simulink model "ctrl_TT_ad_ctrl_cpp_ros_feedback"  (R2022b)
settings: Solver=FixedStepAuto  StartTime=0.0  StopTime=Tf  FixedStep=0.05  RelTol=1e-3
StopFcn:
  | save('testdata')
values from neighbouring files (symbols this model uses):
  adap = 1    [testdata.mat]
  Ba_0 = [0 0 0 0 0 0]    [testdata.mat]
  Bb = 4418825.3321    [testdata.mat]
  Bv_0 = [-5.14444 0 0 0 0 0]    [testdata.mat]
  Bx_0 = [70.34790039 -18.70597267 -370.8000183 0 0 0]    [testdata.mat]
  Cp = [-70.34790039 18.70597267 -370.8000183 -33.25566673 18.72042656 -369.9571533 3.8263092 17.99342728 -368.5174255 40.77630615 14.78142262 -366.2670288 ... (183 elements, 3x61)]    [testdata.mat]    (also in tester.m = [Cpx'; Cpy'; Cpz'])
  Cp_prime = [4.4510680392 0.0017344668 0.1011438 4.44985762706 -0.08575700726 0.1715736104 4.43452754992 -0.37550053768 0.2668049284 4.4276356638 -0.45576590634 0.3213246444 ... (183 elements, 3x61)]    [testdata.mat]
  d = 250    [testdata.mat]
  dA_BP1 = [0.00388591051125 0.00354364911083 0.00553040741788 0.00502167988714 0.0078585088908 0.00748424955325 0.0119232766011 0.0109054787122 0.0168329706434 0.016985509009 0.0156802934897 0.014556760782 ... (616 elements, 616x1)]    [testdata.mat]
  dA_BP2 = [0.00388594063171 0.00354357191533 0.00553040491113 0.00502170939051 0.00785855989083 0.00748435285791 0.0119232653011 0.0109054419481 0.0168329955973 0.0169854794658 0.015680230324 0.0145567225609 ... (616 elements, 616x1)]    [testdata.mat]
  dA_Hull = [0.896301676511 0.898896720864 0.884294141897 0.886832830172 0.870887902011 0.873360353662 0.856223658523 0.858613244346 0.840314828191 0.842595287849 0.823129385532 0.8253007603 ... (2914 elements, 2914x1)]    [testdata.mat]
  dA_PH = [0.00917454029683 0.00917454029683 0.00646521761836 0.00644666811643 0.011728531678 0.0107683420972 0.0165186720105 0.0100399866209 0.0121147162203 0.00917369783051 0.00917369783051 0.00646462373197 ... (550 elements, 550x1)]    [testdata.mat]
  dA_Sail = [0.08073747293 0.0655437895785 0.0678199581962 0.211496702297 0.185444652254 0.10949647106 0.0763960001413 0.0735864235671 0.0440728222699 0.281106392154 0.32735958292 0.104041938486 ... (564 elements, 564x1)]    [testdata.mat]
  dA_SProot = [0.0225345452169 0.0247277274893 0.0225345452169 0.0480467976325 0.0166447079844 0.0410754287554 0.0247277274893 0.0480467976325 0.0468898715351 0.0839833312794 0.0166447079844 0.0255016718 ... (904 elements, 904x1)]    [testdata.mat]
  dA_X1a = [0.0149621011817 0.0166706156701 0.0341149781095 0.0355915100668 0.0512235531199 0.0489176133683 0.0604458424392 0.0503279152264 0.0577124835488 0.0401555322121 0.044833653096 0.0251568218541 ... (200 elements, 200x1)]    [testdata.mat]
  dA_X1b = [0.0149621011817 0.0166706156701 0.0341149781095 0.0355915100668 0.0512235531199 0.0489176133683 0.0604458424392 0.0503279152264 0.0577124835488 0.0401555322121 0.044833653096 0.0251568218541 ... (200 elements, 200x1)]    [testdata.mat]
  dA_X2a = [0.0149620639393 0.0166705502855 0.0341150948266 0.0355913495849 0.051223110376 0.0489180393921 0.0604458270347 0.0503275686692 0.0577128112225 0.0401556683139 0.0448334591683 0.0251566482124 ... (200 elements, 200x1)]    [testdata.mat]
  dA_X2b = [0.0149620639393 0.0166705502855 0.0341150948266 0.0355913495849 0.051223110376 0.0489180393921 0.0604458270347 0.0503275686692 0.0577128112225 0.0401556683139 0.0448334591683 0.0251566482124 ... (200 elements, 200x1)]    [testdata.mat]
  dA_X3a = [0.0149621011817 0.0166706156701 0.0341149781095 0.0355915100668 0.0512235531199 0.0489176133683 0.0604458424392 0.0503279152264 0.0577124835488 0.0401555322121 0.044833653096 0.0251568218541 ... (200 elements, 200x1)]    [testdata.mat]
  dA_X3b = [0.0149621011817 0.0166706156701 0.0341149781095 0.0355915100668 0.0512235531199 0.0489176133683 0.0604458424392 0.0503279152264 0.0577124835488 0.0401555322121 0.044833653096 0.0251568218541 ... (200 elements, 200x1)]    [testdata.mat]
  dA_X4a = [0.0149621011817 0.0166706156701 0.0341149781095 0.0355915100668 0.0512235531199 0.0489176133683 0.0604458424392 0.0503279152264 0.0577124835488 0.0401555322121 0.044833653096 0.0251568218541 ... (200 elements, 200x1)]    [testdata.mat]
  dA_X4b = [0.0149621011817 0.0166706156701 0.0341149781095 0.0355915100668 0.0512235531199 0.0489176133683 0.0604458424392 0.0503279152264 0.0577124835488 0.0401555322121 0.044833653096 0.0251568218541 ... (200 elements, 200x1)]    [testdata.mat]
  Ixx = 52300000    [testdata.mat]
  Ixy = 0    [testdata.mat]
  Ixz = 0    [testdata.mat]
  Iyy = 1375000000    [testdata.mat]
  Iyz = 0    [testdata.mat]
  Izz = 1367000000    [testdata.mat]
  Kp = 0.1    [testdata.mat]
  L1 =     [testdata.mat]
  Mb = 4418825.3321    [testdata.mat]
  n_BP1 = [-0.7747315 -0.03638153 -0.4095958 0 -0.1221389 0 -0.01670914 0 0.005209626 0 0.03404154 0 ... (1848 elements, 616x3)]    [testdata.mat]
  n_BP2 = [-0.774731517 -0.0363815315 -0.409595788 0 -0.122138903 0 -0.0167091396 0 0.00520962616 0 0.0340415388 0 ... (1848 elements, 616x3)]    [testdata.mat]
  n_Hull = [-3.334458e-05 -1.700098e-14 -3.354233e-05 -1.686235e-14 -3.289162e-05 -1.685701e-14 -3.291391e-05 -1.698144e-14 -3.338145e-05 -1.688959e-14 -3.29289e-05 -1.682536e-14 ... (8742 elements, 2914x3)]    [testdata.mat]
  n_PH = [0 0 0.01711651 0.01711627 0.2676807 0.2676804 0.7675173 0.7675174 0.9857236 0 0 0.01711456 ... (1650 elements, 550x3)]    [testdata.mat]
  n_Sail = [-0.05126832 -0.05168081 -0.0485872 -0.03288998 -0.03203588 -0.04435105 -0.04335441 -0.04419429 -0.05169604 0.01094904 0.01649325 -0.03825178 ... (1692 elements, 564x3)]    [testdata.mat]
  n_SProot = [-0.7837688 -0.7969784 -0.7837688 -0.79448 -0.280412 -0.3378876 -0.7969784 -0.79448 -0.7910827 -0.3483897 -0.280412 -0.2790298 ... (2712 elements, 904x3)]    [testdata.mat]
  n_X2a = [-0.283297986 -0.283136904 -0.283195704 -0.28313759 -0.2831586 -0.283137113 -0.28313911 -0.283136606 -0.283121586 -0.283136815 -0.283108413 -0.283138901 ... (600 elements, 200x3)]    [testdata.mat]
  n_X2b = [-0.283297986 -0.283136904 -0.283195704 -0.28313759 -0.2831586 -0.283137113 -0.28313911 -0.283136606 -0.283121586 -0.283136815 -0.283108413 -0.283138901 ... (600 elements, 200x3)]    [testdata.mat]
  n_X3a = [-0.283298 -0.2831369 -0.2831957 -0.2831376 -0.2831586 -0.2831371 -0.2831391 -0.2831366 -0.2831216 -0.2831368 -0.2831084 -0.2831389 ... (600 elements, 200x3)]    [testdata.mat]
  n_X4a = [-0.283298 -0.2831369 -0.2831957 -0.2831376 -0.2831586 -0.2831371 -0.2831391 -0.2831366 -0.2831216 -0.2831368 -0.2831084 -0.2831389 ... (600 elements, 200x3)]    [testdata.mat]
  n_X4b = [-0.283298 -0.2831369 -0.2831957 -0.2831376 -0.2831586 -0.2831371 -0.2831391 -0.2831366 -0.2831216 -0.2831368 -0.2831084 -0.2831389 ... (600 elements, 200x3)]    [testdata.mat]
  nt_BP1 = 616    [testdata.mat]
  nt_BP2 = 616    [testdata.mat]
  nt_Hull = 2914    [testdata.mat]
  nt_PH = 550    [testdata.mat]
  nt_Sail = 564    [testdata.mat]
  nt_SProot = 904    [testdata.mat]
  nt_X1a = 200    [testdata.mat]
  nt_X1b = 200    [testdata.mat]
  nt_X2a = 200    [testdata.mat]
  nt_X2b = 200    [testdata.mat]
  nt_X3a = 200    [testdata.mat]
  nt_X3b = 200    [testdata.mat]
  nt_X4a = 200    [testdata.mat]
  nt_X4b = 200    [testdata.mat]
  Seastate = 0    [testdata.mat]
  Tf = 500    [testdata.mat]    (also in tester.m)
  Ts = 0.05    [testdata.mat]
  vt1_BP1 = [-11.0524049722 -10.9924120522 -10.9924120522 -10.8819663922 -10.8819663922 -10.7297166322 -10.7297166322 -10.5070632922 -10.5070632922 -10.1807245522 -10.1807245522 -9.8815181122 ... (1848 elements, 616x3)]    [testdata.mat]
  vt1_BP2 = [-11.0524048318 -10.9924111396 -10.9924111396 -10.8819658306 -10.8819658306 -10.7297157898 -10.7297157898 -10.5070637134 -10.5070637134 -10.1807238502 -10.1807238502 -9.8815188844 ... (1848 elements, 616x3)]    [testdata.mat]
  vt1_Hull = [3.5122487678 3.7304022878 5.2621803278 5.4863499878 6.9866994878 7.2167238278 8.6832650078 8.9189474678 10.3493567078 10.5904445678 11.9823842078 12.2286247478 ... (8742 elements, 2914x3)]    [testdata.mat]
  vt1_PH = [37.3342788278 37.3342788278 37.4268866678 37.4268866678 37.5892452278 37.5892452278 37.7549453078 37.7549453078 37.8074619278 37.3342788278 37.3342788278 37.4268866678 ... (1650 elements, 550x3)]    [testdata.mat]
  vt1_Sail = [-12.4909433722 -12.1578443722 -12.0399645322 -11.2138368922 -10.6240515922 -11.5111900522 -11.9364967522 -11.6561249722 -12.4909433722 -7.5732648922 -6.8453119522 -11.1890071522 ... (1692 elements, 564x3)]    [testdata.mat]
  vt1_SProot = [29.2099766678 29.1371231078 29.0494854278 29.2099766678 29.2862630078 29.4526510478 29.0494854278 29.1261368078 29.3369263478 29.5706712878 29.0494854278 29.3857364078 ... (2712 elements, 904x3)]    [testdata.mat]
  vt1_X1a = [29.3961751478 29.4776282078 29.4776282078 29.7060309278 29.7060309278 30.0693861278 30.0693861278 30.5458756478 30.5458756478 31.0830460478 31.0830460478 31.6023926678 ... (600 elements, 200x3)]    [testdata.mat]
  vt1_X1b = [29.6638337078 29.6638337078 29.9620713878 29.9620713878 30.3181187678 30.3181187678 30.7116389078 30.7116389078 31.1104380878 31.1104380878 31.4810519678 31.4810519678 ... (600 elements, 200x3)]    [testdata.mat]
  vt1_X2a = [29.3961767624 29.4776272952 29.4776272952 29.7060326828 29.7060326828 30.0693842324 30.0693842324 30.5458736822 30.5458736822 31.083047171 31.083047171 31.6023916148 ... (600 elements, 200x3)]    [testdata.mat]
  vt1_X2b = [29.6638345502 29.6638345502 29.9620708964 29.9620708964 30.3181168022 30.3181168022 30.7116409436 30.7116409436 31.1104372454 31.1104372454 31.4810526698 31.4810526698 ... (600 elements, 200x3)]    [testdata.mat]
  vt1_X3a = [29.3961751478 29.4776282078 29.4776282078 29.7060309278 29.7060309278 30.0693861278 30.0693861278 30.5458756478 30.5458756478 31.0830460478 31.0830460478 31.6023926678 ... (600 elements, 200x3)]    [testdata.mat]
  vt1_X3b = [29.6638337078 29.6638337078 29.9620713878 29.9620713878 30.3181187678 30.3181187678 30.7116389078 30.7116389078 31.1104380878 31.1104380878 31.4810519678 31.4810519678 ... (600 elements, 200x3)]    [testdata.mat]
  vt1_X4a = [29.6638337078 29.6638337078 29.9620713878 29.9620713878 30.3181187678 30.3181187678 30.7116389078 30.7116389078 31.1104380878 31.1104380878 31.4810519678 31.4810519678 ... (600 elements, 200x3)]    [testdata.mat]
  vt1_X4b = [29.3961751478 29.4776282078 29.4776282078 29.7060309278 29.7060309278 30.0693861278 30.0693861278 30.5458756478 30.5458756478 31.0830460478 31.0830460478 31.6023926678 ... (600 elements, 200x3)]    [testdata.mat]
  vt2_BP1 = [-10.9924120522 -10.9494777322 -10.8819663922 -10.8505308322 -10.7297166322 -10.7112259522 -10.5070632922 -10.4997203722 -10.1807245522 -10.1757543922 -9.8815181122 -9.8813004922 ... (1848 elements, 616x3)]    [testdata.mat]
  vt2_BP2 = [-11.0294626294 -11.0294626294 -10.9494786448 -10.9494786448 -10.8505316746 -10.8505316746 -10.7112256012 -10.7112256012 -10.499720302 -10.499720302 -10.1757550942 -10.1757550942 ... (1848 elements, 616x3)]    [testdata.mat]
  vt2_Hull = [1.9517168078 1.9517168078 3.7304022878 3.7304022878 5.4863499878 5.4863499878 7.2167238278 7.2167238278 8.9189474678 8.9189474678 10.5904445678 10.5904445678 ... (8742 elements, 2914x3)]    [testdata.mat]
  vt2_PH = [37.2028433678 37.2028433678 37.3342788278 37.4268866678 37.4268866678 37.5892452278 37.5892452278 37.7549453078 37.7549453078 37.2028433678 37.2028433678 37.3342788278 ... (1650 elements, 550x3)]    [testdata.mat]
  vt2_Sail = [-12.0399645322 -12.0399645322 -11.9364967522 -10.7084881522 -10.7084881522 -12.0399645322 -12.0399645322 -11.9364967522 -12.3734566522 -7.7110323922 -7.7110323922 -11.6561249722 ... (1692 elements, 564x3)]    [testdata.mat]
  vt2_SProot = [29.0494854278 29.0494854278 29.2099766678 29.1261368078 29.0494854278 29.1371231078 29.1371231078 29.2099766678 29.1261368078 29.2099766678 29.2862630078 29.2862630078 ... (2712 elements, 904x3)]    [testdata.mat]
  vt2_X1a = [29.4776282078 29.9620713878 29.7060309278 30.3181187678 30.0693861278 30.7116389078 30.5458756478 31.1104380878 31.0830460478 31.4810519678 31.6023926678 31.7970362078 ... (600 elements, 200x3)]    [testdata.mat]
  vt2_X1b = [29.4776282078 29.9620713878 29.7060309278 30.3181187678 30.0693861278 30.7116389078 30.5458756478 31.1104380878 31.0830460478 31.4810519678 31.6023926678 31.7970362078 ... (600 elements, 200x3)]    [testdata.mat]
  vt2_X2a = [29.6638345502 29.6638345502 29.9620708964 29.9620708964 30.3181168022 30.3181168022 30.7116409436 30.7116409436 31.1104372454 31.1104372454 31.4810526698 31.4810526698 ... (600 elements, 200x3)]    [testdata.mat]
  vt2_X2b = [29.3961767624 29.4776272952 29.4776272952 29.7060326828 29.7060326828 30.0693842324 30.0693842324 30.5458736822 30.5458736822 31.083047171 31.083047171 31.6023916148 ... (600 elements, 200x3)]    [testdata.mat]
  vt2_X3a = [29.4776282078 29.9620713878 29.7060309278 30.3181187678 30.0693861278 30.7116389078 30.5458756478 31.1104380878 31.0830460478 31.4810519678 31.6023926678 31.7970362078 ... (600 elements, 200x3)]    [testdata.mat]
  vt2_X3b = [29.4776282078 29.9620713878 29.7060309278 30.3181187678 30.0693861278 30.7116389078 30.5458756478 31.1104380878 31.0830460478 31.4810519678 31.6023926678 31.7970362078 ... (600 elements, 200x3)]    [testdata.mat]
  vt2_X4a = [29.4776282078 29.9620713878 29.7060309278 30.3181187678 30.0693861278 30.7116389078 30.5458756478 31.1104380878 31.0830460478 31.4810519678 31.6023926678 31.7970362078 ... (600 elements, 200x3)]    [testdata.mat]
  vt2_X4b = [29.4776282078 29.9620713878 29.7060309278 30.3181187678 30.0693861278 30.7116389078 30.5458756478 31.1104380878 31.0830460478 31.4810519678 31.6023926678 31.7970362078 ... (600 elements, 200x3)]    [testdata.mat]
  vt3_BP1 = [-11.0294636122 -11.0294636122 -10.9494777322 -10.9494777322 -10.8505308322 -10.8505308322 -10.7112259522 -10.7112259522 -10.4997203722 -10.4997203722 -10.1757543922 -10.1757543922 ... (1848 elements, 616x3)]    [testdata.mat]
  vt3_BP2 = [-10.9924111396 -10.9494786448 -10.8819658306 -10.8505316746 -10.7297157898 -10.7112256012 -10.5070637134 -10.499720302 -10.1807238502 -10.1757550942 -9.8815188844 -9.8813013346 ... (1848 elements, 616x3)]    [testdata.mat]
  vt3_Hull = [1.7397198278 3.5122487678 3.5122487678 5.2621803278 5.2621803278 6.9866994878 6.9866994878 8.6832650078 8.6832650078 10.3493567078 10.3493567078 11.9823842078 ... (8742 elements, 2914x3)]    [testdata.mat]
  vt3_PH = [37.2028433678 37.3342788278 37.3342788278 37.3342788278 37.4268866678 37.4268866678 37.5892452278 37.5892452278 37.7549453078 37.2028433678 37.3342788278 37.3342788278 ... (1650 elements, 550x3)]    [testdata.mat]
  vt3_Sail = [-12.3734566522 -12.4909433722 -12.3734566522 -11.5111900522 -11.2138368922 -11.7698559922 -11.5111900522 -11.5111900522 -12.1578443722 -8.3109054322 -7.5732648922 -11.5111900522 ... (1692 elements, 564x3)]    [testdata.mat]
  vt3_SProot = [29.1261368078 29.2099766678 29.1261368078 29.3369263478 29.1371231078 29.2099766678 29.2099766678 29.3369263478 29.2548344678 29.3369263478 29.1371231078 29.1371231078 ... (2712 elements, 904x3)]    [testdata.mat]
  vt3_X1a = [29.6638337078 29.6638337078 29.9620713878 29.9620713878 30.3181187678 30.3181187678 30.7116389078 30.7116389078 31.1104380878 31.1104380878 31.4810519678 31.4810519678 ... (600 elements, 200x3)]    [testdata.mat]
  vt3_X1b = [29.3961751478 29.4776282078 29.4776282078 29.7060309278 29.7060309278 30.0693861278 30.0693861278 30.5458756478 30.5458756478 31.0830460478 31.0830460478 31.6023926678 ... (600 elements, 200x3)]    [testdata.mat]
  vt3_X2a = [29.4776272952 29.9620708964 29.7060326828 30.3181168022 30.0693842324 30.7116409436 30.5458736822 31.1104372454 31.083047171 31.4810526698 31.6023916148 31.7970343826 ... (600 elements, 200x3)]    [testdata.mat]
  vt3_X2b = [29.4776272952 29.9620708964 29.7060326828 30.3181168022 30.0693842324 30.7116409436 30.5458736822 31.1104372454 31.083047171 31.4810526698 31.6023916148 31.7970343826 ... (600 elements, 200x3)]    [testdata.mat]
  vt3_X3a = [29.6638337078 29.6638337078 29.9620713878 29.9620713878 30.3181187678 30.3181187678 30.7116389078 30.7116389078 31.1104380878 31.1104380878 31.4810519678 31.4810519678 ... (600 elements, 200x3)]    [testdata.mat]
  vt3_X3b = [29.3961751478 29.4776282078 29.4776282078 29.7060309278 29.7060309278 30.0693861278 30.0693861278 30.5458756478 30.5458756478 31.0830460478 31.0830460478 31.6023926678 ... (600 elements, 200x3)]    [testdata.mat]
  vt3_X4a = [29.3961751478 29.4776282078 29.4776282078 29.7060309278 29.7060309278 30.0693861278 30.0693861278 30.5458756478 30.5458756478 31.0830460478 31.0830460478 31.6023926678 ... (600 elements, 200x3)]    [testdata.mat]
  vt3_X4b = [29.6638337078 29.6638337078 29.9620713878 29.9620713878 30.3181187678 30.3181187678 30.7116389078 30.7116389078 31.1104380878 31.1104380878 31.4810519678 31.4810519678 ... (600 elements, 200x3)]    [testdata.mat]
  Xb = 0    [testdata.mat]
  Xcg = [32.3287332922 0 0]    [testdata.mat]
  Xg = 0    [testdata.mat]
  Yb = 0    [testdata.mat]
  Yg = 0    [testdata.mat]
  Zb = 0.4406    [testdata.mat]
  Zg = 0    [testdata.mat]
libraries: robotlib x54, simulink x8, sharedtransform x2, dspmathops x2
(part 1 of 9)
settings Model: Creator=yagkim  LastModifiedBy=vpetrov
settings SolverCC: AlgebraicLoopSolver=TrustRegion
settings OptimizationCC: EnhancedBackFolding=on  PassReuseOutputArgsAs=Individual arguments  ZeroExternalMemoryAtStartup=off  ZeroInternalMemoryAtStartup=off  MaxStackSize=64  OptimizeBlockOrder=speed  DifferentSizesBufferReuse=on  OptimizationCustomize=off  EfficientTunableParamExpr=on
settings DebuggingCC: ParameterTunabilityLossMsg=error  UnconnectedInputMsg=warning  UnconnectedOutputMsg=warning  UnconnectedLineMsg=warning  SFMachineParentedDataDiag=warning  ArithmeticOperatorsInVariantConditions=warning
settings HardwareCC: ProdBitPerPointer=32  ProdBitPerSizeT=32  ProdBitPerPtrDiffT=32  ProdLargestAtomicFloat=None  ProdIntDivRoundTo=Undefined  ProdEndianess=Unspecified  ProdWordSize=32  ProdHWDeviceType=Generic->Unspecified (assume 32-bit Generic)
settings ModelReferenceCC: EnableRefExpFcnMdlSchedulingChecks=on
settings SFSimCC: MATLABDynamicMemAlloc=off  CustomCodeUndefinedFunction=UseInterfaceOnly  SimTargetLang=C++
settings RTWCC: Description=Embedded Coder  SystemTargetFile=ert.tlc  HardwareBoard=Robot Operating System (ROS)  TLCOptions="-aInlineSetEventsForThisBaseRateFcn=TLC_FALSE -aSuppressMultiTaskScheduler=TLC_FALSE  -aRateBasedStepFcn=0"  TemplateMakefile=ert_default_tmf  GenerateReport=on  Toolchain=Catkin  LaunchReport=on  TargetLang=C++  DLArmComputeVersion=19.05
settings CodeAppCC: ForceParamTrailComments=on  IgnoreCustomStorageClasses=off  OperatorAnnotations=on  SimulinkDataObjDesc=on  SFDataObjDesc=on  InsertBlockDesc=on
settings ERTTargetCC: SupportContinuousTime=on

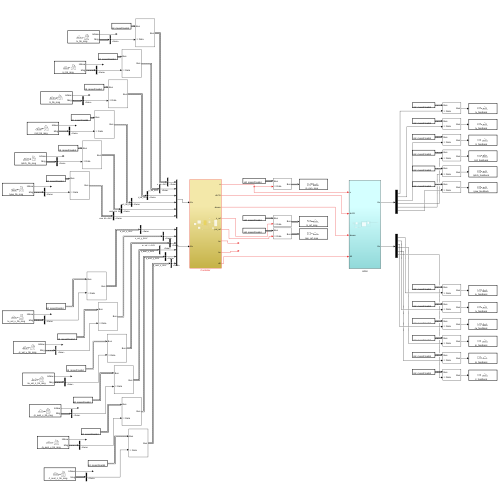
[thumbnail: Simulink's stored preview of the top-level diagram]
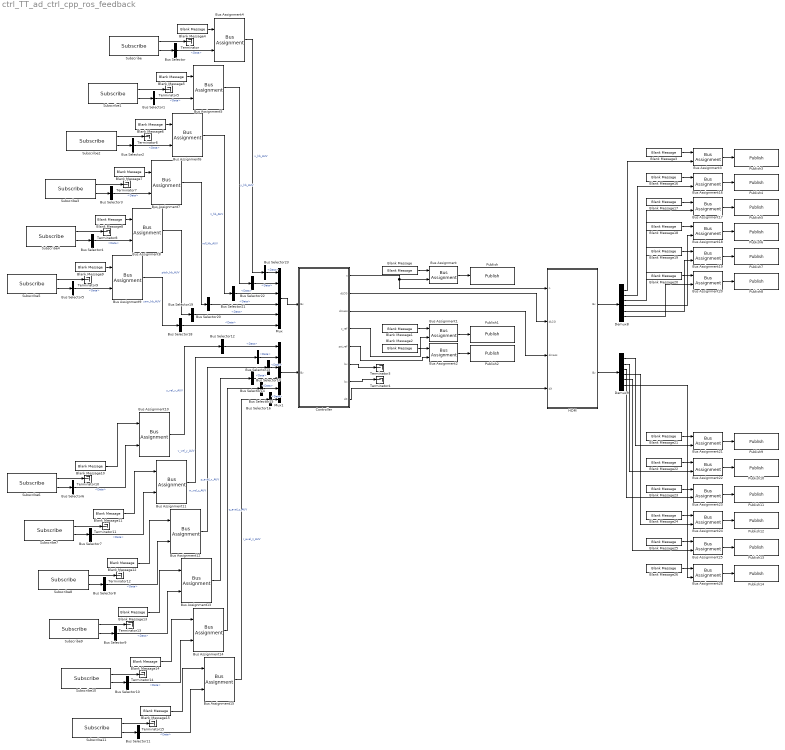
== system ctrl_TT_ad_ctrl_cpp_ros_feedback ==
  Blank Message{,1..26} (27 alike) : robotlib/Blank Message  messageClass=Message  entityType=std_msgs/Float64  messageType=std_msgs/Float64  SampleTime=inf  legacyBusStruct=off
      settings: LibrarySourceBlock=roslib/ROS/Blank Message
  Bus Assignment{,1..26} (27 alike) : BusAssignment  AssignedSignals=Data
  Bus Selector{,1..23} (24 alike) : BusSelector  OutputSignals=Data
  Controller : Subsystem
  Demux8 : Demux  Outputs=6
  Demux9 : Demux  Outputs=6
  HDM : Subsystem
  Mux : Mux  Inputs=6
  Mux1 : Mux  Inputs=6
  Publish : robotlib/Publish  topicSource=Specify your own  topic=/n_rpm_msg  messageType=std_msgs/Float64  legacyBusStruct=off  messageQueueLength=1
      settings: LibrarySourceBlock=roslib/ROS/Publish
  Publish1 : robotlib/Publish  topicSource=Specify your own  topic=/z_ref_msg  messageType=std_msgs/Float64  legacyBusStruct=off  messageQueueLength=1
      settings: LibrarySourceBlock=roslib/ROS/Publish
  Publish10 : robotlib/Publish  topicSource=Specify your own  topic=/v_feedback  messageType=std_msgs/Float64  legacyBusStruct=off  messageQueueLength=1
      settings: LibrarySourceBlock=roslib/ROS/Publish
  Publish11 : robotlib/Publish  topicSource=Specify your own  topic=/w_feedback  messageType=std_msgs/Float64  legacyBusStruct=off  messageQueueLength=1
      settings: LibrarySourceBlock=roslib/ROS/Publish
  Publish12 : robotlib/Publish  topicSource=Specify your own  topic=/p_feedback  messageType=std_msgs/Float64  legacyBusStruct=off  messageQueueLength=1
      settings: LibrarySourceBlock=roslib/ROS/Publish
  Publish13 : robotlib/Publish  topicSource=Specify your own  topic=/q_feedback  messageType=std_msgs/Float64  legacyBusStruct=off  messageQueueLength=1
      settings: LibrarySourceBlock=roslib/ROS/Publish
  Publish14 : robotlib/Publish  topicSource=Specify your own  topic=/r_feedback  messageType=std_msgs/Float64  legacyBusStruct=off  messageQueueLength=1
      settings: LibrarySourceBlock=roslib/ROS/Publish
  Publish2 : robotlib/Publish  topicSource=Specify your own  topic=/psi_ref_msg  messageType=std_msgs/Float64  legacyBusStruct=off  messageQueueLength=1
      settings: LibrarySourceBlock=roslib/ROS/Publish
  Publish3 : robotlib/Publish  topicSource=Specify your own  topic=/x_feedback  messageType=std_msgs/Float64  legacyBusStruct=off  messageQueueLength=1
      settings: LibrarySourceBlock=roslib/ROS/Publish
  Publish4 : robotlib/Publish  topicSource=Specify your own  topic=/y_feedback  messageType=std_msgs/Float64  legacyBusStruct=off  messageQueueLength=1
      settings: LibrarySourceBlock=roslib/ROS/Publish
  Publish5 : robotlib/Publish  topicSource=Specify your own  topic=/z_feedback  messageType=std_msgs/Float64  legacyBusStruct=off  messageQueueLength=1
      settings: LibrarySourceBlock=roslib/ROS/Publish
  Publish6 : robotlib/Publish  topicSource=Specify your own  topic=/roll_feedback  messageType=std_msgs/Float64  legacyBusStruct=off  messageQueueLength=1
      settings: LibrarySourceBlock=roslib/ROS/Publish
  Publish7 : robotlib/Publish  topicSource=Specify your own  topic=/pitch_feedback  messageType=std_msgs/Float64  legacyBusStruct=off  messageQueueLength=1
      settings: LibrarySourceBlock=roslib/ROS/Publish
  Publish8 : robotlib/Publish  topicSource=Specify your own  topic=/yaw_feedback  messageType=std_msgs/Float64  legacyBusStruct=off  messageQueueLength=1
      settings: LibrarySourceBlock=roslib/ROS/Publish
  Publish9 : robotlib/Publish  topicSource=Specify your own  topic=/u_feedback  messageType=std_msgs/Float64  legacyBusStruct=off  messageQueueLength=1
      settings: LibrarySourceBlock=roslib/ROS/Publish
  Subscribe : robotlib/Subscribe  topicSource=Specify your own  topic=/x_hb_msg  messageType=std_msgs/Float64  SampleTime=-1  legacyBusStruct=off  messageQueueLength=1
      settings: LibrarySourceBlock=roslib/ROS/Subscribe
  Subscribe1 : robotlib/Subscribe  topicSource=Specify your own  topic=/y_hb_msg  messageType=std_msgs/Float64  SampleTime=-1  legacyBusStruct=off  messageQueueLength=1
      settings: LibrarySourceBlock=roslib/ROS/Subscribe
  Subscribe10 : robotlib/Subscribe  topicSource=Specify your own  topic=/q_avel_y_hb_msg  messageType=std_msgs/Float64  SampleTime=-1  legacyBusStruct=off  messageQueueLength=1
      settings: LibrarySourceBlock=roslib/ROS/Subscribe
  Subscribe11 : robotlib/Subscribe  topicSource=Specify your own  topic=/r_avel_z_hb_msg  messageType=std_msgs/Float64  SampleTime=-1  legacyBusStruct=off  messageQueueLength=1
      settings: LibrarySourceBlock=roslib/ROS/Subscribe
  Subscribe2 : robotlib/Subscribe  topicSource=Specify your own  topic=/z_hb_msg  messageType=std_msgs/Float64  SampleTime=-1  legacyBusStruct=off  messageQueueLength=1
      settings: LibrarySourceBlock=roslib/ROS/Subscribe
  Subscribe3 : robotlib/Subscribe  topicSource=Specify your own  topic=/roll_hb_msg  messageType=std_msgs/Float64  SampleTime=-1  legacyBusStruct=off  messageQueueLength=1
      settings: LibrarySourceBlock=roslib/ROS/Subscribe
  Subscribe4 : robotlib/Subscribe  topicSource=Specify your own  topic=/pitch_hb_msg  messageType=std_msgs/Float64  SampleTime=-1  legacyBusStruct=off  messageQueueLength=1
      settings: LibrarySourceBlock=roslib/ROS/Subscribe
  Subscribe5 : robotlib/Subscribe  topicSource=Specify your own  topic=/yaw_hb_msg  messageType=std_msgs/Float64  SampleTime=-1  legacyBusStruct=off  messageQueueLength=1
      settings: LibrarySourceBlock=roslib/ROS/Subscribe
  Subscribe6 : robotlib/Subscribe  topicSource=Specify your own  topic=/u_vel_x_hb_msg  messageType=std_msgs/Float64  SampleTime=-1  legacyBusStruct=off  messageQueueLength=1
      settings: LibrarySourceBlock=roslib/ROS/Subscribe
  Subscribe7 : robotlib/Subscribe  topicSource=Specify your own  topic=/v_vel_y_hb_msg  messageType=std_msgs/Float64  SampleTime=-1  legacyBusStruct=off  messageQueueLength=1
      settings: LibrarySourceBlock=roslib/ROS/Subscribe
  Subscribe8 : robotlib/Subscribe  topicSource=Specify your own  topic=/w_vel_z_hb_msg  messageType=std_msgs/Float64  SampleTime=-1  legacyBusStruct=off  messageQueueLength=1
      settings: LibrarySourceBlock=roslib/ROS/Subscribe
  Subscribe9 : robotlib/Subscribe  topicSource=Specify your own  topic=/p_avel_x_hb_msg  messageType=std_msgs/Float64  SampleTime=-1  legacyBusStruct=off  messageQueueLength=1
      settings: LibrarySourceBlock=roslib/ROS/Subscribe
  Terminator{,3..15} (14 alike) : Terminator
  wires:
  Bus Assignment4/1 -> Bus Selector23/1  "x_hb_AUV"
  Bus Assignment6/1 -> Bus Selector21/1  "z_hb_AUV"
  Bus Assignment7/1 -> Bus Selector20/1  "roll_hb_AUV"
  Bus Assignment8/1 -> Bus Selector19/1  "pitch_hb_AUV"
  Bus Assignment9/1 -> Bus Selector18/1  "yaw_hb_AUV"
  Mux/1 -> Controller/1(Bx)
  Mux1/1 -> Controller/2(Bv)
  Bus Assignment11/1 -> Bus Selector13/1  "v_vel_y_AUV"
  Bus Assignment12/1 -> Bus Selector17/1  "w_vel_z_AUV"
  Bus Assignment13/1 -> Bus Selector14/1  "p_avel_x_AUV"
  Bus Assignment14/1 -> Bus Selector15/1  "q_avel_y_AUV"
  Bus Assignment15/1 -> Bus Selector16/1  "r_avel_z_AUV"
  Controller/2(dLCG) -> HDM/2(dLCG)
  Controller/3(dmass) -> HDM/3(dmass)
  Controller/1(n) -> Bus Assignment/2, HDM/1(n)
  Controller/4(z_ref) -> Bus Assignment1/2
  Controller/5(psi_ref) -> Bus Assignment2/2
  Controller/6(bv) -> Terminator3/1
  Controller/7(bx) -> Terminator4/1
  Bus Assignment/1 -> Publish/1
  Blank Message/1 -> Bus Assignment/1
  Blank Message1/1 -> Bus Assignment1/1
  Bus Assignment1/1 -> Publish1/1
  Blank Message2/1 -> Bus Assignment2/1
  Bus Assignment2/1 -> Publish2/1
  Subscribe/1 -> Terminator/1
  Bus Selector/1 -> Bus Assignment4/2  "<Data>"
  Subscribe/2 -> Bus Selector/1
  Blank Message4/1 -> Bus Assignment4/1
  Subscribe1/1 -> Terminator5/1
  Bus Selector1/1 -> Bus Assignment5/2  "<Data>"
  Blank Message5/1 -> Bus Assignment5/1
  Subscribe1/2 -> Bus Selector1/1
  Bus Assignment5/1 -> Bus Selector22/1  "y_hb_AUV"
  Blank Message6/1 -> Bus Assignment6/1
  Bus Selector2/1 -> Bus Assignment6/2  "<Data>"
  Subscribe2/2 -> Bus Selector2/1
  Subscribe2/1 -> Terminator6/1
  Blank Message7/1 -> Bus Assignment7/1
  Bus Selector3/1 -> Bus Assignment7/2  "<Data>"
  Subscribe3/2 -> Bus Selector3/1
  Subscribe3/1 -> Terminator7/1
  Blank Message8/1 -> Bus Assignment8/1
  Bus Selector4/1 -> Bus Assignment8/2  "<Data>"
  Subscribe4/2 -> Bus Selector4/1
  Subscribe4/1 -> Terminator8/1
  Bus Selector5/1 -> Bus Assignment9/2  "<Data>"
  Subscribe5/2 -> Bus Selector5/1
  Blank Message9/1 -> Bus Assignment9/1
  Subscribe5/1 -> Terminator9/1
  Bus Selector6/1 -> Bus Assignment10/2  "<Data>"
  Subscribe6/2 -> Bus Selector6/1
  Blank Message10/1 -> Bus Assignment10/1
  Subscribe6/1 -> Terminator10/1
  Bus Assignment10/1 -> Bus Selector12/1  "u_vel_x_AUV"
  Bus Selector7/1 -> Bus Assignment11/2  "<Data>"
  Blank Message11/1 -> Bus Assignment11/1
  Subscribe7/2 -> Bus Selector7/1
  Subscribe7/1 -> Terminator11/1
  Bus Selector8/1 -> Bus Assignment12/2  "<Data>"
  Blank Message12/1 -> Bus Assignment12/1
  Subscribe8/2 -> Bus Selector8/1
  Subscribe8/1 -> Terminator12/1
  Bus Selector9/1 -> Bus Assignment13/2  "<Data>"
  Blank Message13/1 -> Bus Assignment13/1
  Subscribe9/2 -> Bus Selector9/1
  Subscribe9/1 -> Terminator13/1
  Bus Selector10/1 -> Bus Assignment14/2  "<Data>"
  Blank Message14/1 -> Bus Assignment14/1
  Subscribe10/2 -> Bus Selector10/1
  Subscribe10/1 -> Terminator14/1
  Bus Selector11/1 -> Bus Assignment15/2  "<Data>"
  Blank Message15/1 -> Bus Assignment15/1
  Subscribe11/2 -> Bus Selector11/1
  Subscribe11/1 -> Terminator15/1
  Bus Selector12/1 -> Mux1/1  "<Data>"
  Bus Selector13/1 -> Mux1/2  "<Data>"
  Bus Selector14/1 -> Mux1/4  "<Data>"
  Bus Selector15/1 -> Mux1/5  "<Data>"
  Bus Selector16/1 -> Mux1/6  "<Data>"
  Bus Selector17/1 -> Mux1/3  "<Data>"
  Bus Selector18/1 -> Mux/6  "<Data>"
  Bus Selector19/1 -> Mux/5  "<Data>"
  Bus Selector20/1 -> Mux/4  "<Data>"
  Bus Selector21/1 -> Mux/3  "<Data>"
  Bus Selector22/1 -> Mux/2  "<Data>"
  Bus Selector23/1 -> Mux/1  "<Data>"
  Controller/8(dX) -> HDM/4(dX)
  HDM/1(Bx) -> Demux8/1
  HDM/2(Bv) -> Demux9/1
  Blank Message3/1 -> Bus Assignment3/1
  Demux8/1 -> Bus Assignment3/2
  Bus Assignment3/1 -> Publish3/1
  Bus Assignment16/1 -> Publish4/1
  Demux8/2 -> Bus Assignment16/2
  Blank Message16/1 -> Bus Assignment16/1
  Bus Assignment17/1 -> Publish5/1
  Demux8/3 -> Bus Assignment17/2
  Blank Message17/1 -> Bus Assignment17/1
  Blank Message18/1 -> Bus Assignment18/1
  Bus Assignment18/1 -> Publish6/1
  Blank Message19/1 -> Bus Assignment19/1
  Bus Assignment19/1 -> Publish7/1
  Blank Message20/1 -> Bus Assignment20/1
  Bus Assignment20/1 -> Publish8/1
  Demux8/4 -> Bus Assignment18/2
  Demux8/5 -> Bus Assignment19/2
  Demux8/6 -> Bus Assignment20/2
  Bus Assignment21/1 -> Publish9/1
  Blank Message21/1 -> Bus Assignment21/1
  Bus Assignment22/1 -> Publish10/1
  Blank Message22/1 -> Bus Assignment22/1
  Bus Assignment23/1 -> Publish11/1
  Blank Message23/1 -> Bus Assignment23/1
  Bus Assignment24/1 -> Publish12/1
  Blank Message24/1 -> Bus Assignment24/1
  Bus Assignment25/1 -> Publish13/1
  Blank Message25/1 -> Bus Assignment25/1
  Bus Assignment26/1 -> Publish14/1
  Blank Message26/1 -> Bus Assignment26/1
  Demux9/1 -> Bus Assignment21/2
  Demux9/2 -> Bus Assignment22/2
  Demux9/3 -> Bus Assignment23/2
  Demux9/4 -> Bus Assignment24/2
  Demux9/5 -> Bus Assignment25/2
  Demux9/6 -> Bus Assignment26/2

== system ctrl_TT_ad_ctrl_cpp_ros_feedback/Controller ==
  Bx : Inport
  Bv : Inport  Port=2
  Clock : Clock
  Constant : Constant  Value=[-1 0 0 0 0 0; 0 -1 0 0 0 0; 0 0 1 0 0 0; 0 0 0 1 0 0; 0 0 0 0 1 0; 0 0 0 0 0 1]
  Constant1 : Constant  Value=0
  Constant2 : Constant  Value=[-1 0 0 0 0 0; 0 -1 0 0 0 0; 0 0 1 0 0 0; 0 0 0 1 0 0; 0 0 0 0 1 0; 0 0 0 0 0 1]
  FF velocity ctrl : MATLAB Function  TreatAsAtomicUnit=on
  MATLAB Function2 : MATLAB Function  TreatAsAtomicUnit=on
  Marin PID : MATLAB Function  TreatAsAtomicUnit=on
  Matrix Multiply : Product  Multiplication=Matrix(*)
  Matrix Multiply1 : Product  Multiplication=Matrix(*)
  Selector1 : Selector  InputPortWidth=6  IndexOptions=Index vector (dialog)  Indices=[1 2 3]  OutputSizes=1
  Subsystem1 : Subsystem
  l1 aug - depth : MATLAB Function  TreatAsAtomicUnit=on
  l1 aug - heading : MATLAB Function  TreatAsAtomicUnit=on
  n : Outport
  dLCG : Outport  Port=2
  dmass : Outport  Port=3
  z_ref : Outport  Port=4
  psi_ref : Outport  Port=5
  bv : Outport  Port=6
  bx : Outport  Port=7
  dX : Outport  Port=8
  wires:
  FF velocity ctrl/1(n) -> n/1
  Subsystem1/3(v) -> FF velocity ctrl/1(v_ref)
  Constant1/1 -> dLCG/1, dmass/1
  MATLAB Function2/1(pd) -> Subsystem1/1(pd(t))
  MATLAB Function2/2(pdp) -> Subsystem1/2(pd(t)')
  Bx/1 -> Matrix Multiply/2
  Selector1/1 -> Subsystem1/3(p)
  Clock/1 -> MATLAB Function2/1(time)
  Matrix Multiply/1 -> Selector1/1, l1 aug - depth/3(Bx), Marin PID/4(Bx), bx/1, l1 aug - heading/3(Bx)
  Constant/1 -> Matrix Multiply/1
  Bv/1 -> Matrix Multiply1/2
  Matrix Multiply1/1 -> l1 aug - depth/2(Bv), l1 aug - heading/2(Bv), Marin PID/3(Bv), bv/1
  Constant2/1 -> Matrix Multiply1/1
  l1 aug - depth/1(y_aug) -> Marin PID/1(z_ref), z_ref/1
  l1 aug - heading/1(y_aug) -> Marin PID/2(psi_ref), psi_ref/1
  Subsystem1/1(z_d) -> l1 aug - depth/1(y_ref)
  Subsystem1/2(psi_d) -> l1 aug - heading/1(y_ref)
  Marin PID/1(dX) -> dX/1

== system ctrl_TT_ad_ctrl_cpp_ros_feedback/HDM ==
  n : Inport
  dLCG : Inport  Port=2
  dmass : Inport  Port=3
  dX : Inport  Port=4
  Constant1 : Constant  Value=Seastate
  HDM B3 : Subsystem  InitFcn='main'
  Integration and Coord. Transfrom : Subsystem
  Scope : Scope
  Scope1 : Scope
  actuator saturation : Subsystem
  Bx : Outport
  Bv : Outport  Port=2
  wires:
  actuator saturation/4(dmass (kg)) -> HDM B3/4(dmass), Scope1/1
  actuator saturation/3(dLCG (m)) -> HDM B3/3(dLCG)
  actuator saturation/2(n) -> HDM B3/2(n)
  actuator saturation/1(dX) -> HDM B3/1(dX CTRL)
  dmass/1 -> actuator saturation/4(dmass), Scope/1
  dLCG/1 -> actuator saturation/3(dLCG)
  n/1 -> actuator saturation/2("n ")
  dX/1 -> actuator saturation/1("dX ")
  Constant1/1 -> HDM B3/8(SeaState)
  HDM B3/1(F_hyd) -> Integration and Coord. Transfrom/2(F_hyd)
  Integration and Coord. Transfrom/3(Ba) -> HDM B3/7(Ba)
  Integration and Coord. Transfrom/1("Bx ") -> Bx/1, HDM B3/5(Bx), Integration and Coord. Transfrom/1(Bx)
  Integration and Coord. Transfrom/2(Bv) -> Bv/1, HDM B3/6(Bv)

== system ctrl_TT_ad_ctrl_cpp_ros_feedback/Controller/Subsystem1 ==
  pd(t) : Inport
  pd(t)' : Inport  Port=2
  p : Inport  Port=3
  1,1 : Selector  NumberOfDimensions=2  InputPortWidth=3  IndexOptions=Index vector (dialog),Index vector (dialog)  Indices=1,1  OutputSizes=1,1
  2,1 : Selector  NumberOfDimensions=2  InputPortWidth=3  IndexOptions=Index vector (dialog),Index vector (dialog)  Indices=2,1  OutputSizes=1,1
  Add1 : Sum
  Demux3 : Demux  Outputs=3
  Derivative : Derivative
  Direction Cosine Matrix to Rotation Angles : sharedtransform/Direction Cosine Matrix to Rotation Angles  rotationOrder=ZYX  aMode=aMode  action=None  tolerance=eps(2)
      settings: LibrarySourceBlock=|
      | aerolibtransform2/Direction Cosine Matrix
      | to Rotation Angles
  Display{,1..7} (8 alike) : Display
  Dot Product1 : DotProduct  OutDataTypeStr=Inherit: Inherit via internal rule
  Gain : Gain  Gain=-1
  Gain1 : Gain  Gain=Kp
  MATLAB Function : MATLAB Function  TreatAsAtomicUnit=on
  Matrix Multiply1 : Product  Multiplication=Matrix(*)
  Mux1 : Mux  Inputs=2
  Scope : Scope
  Scope1 : Scope
  Selector : Selector  InputPortWidth=3  IndexOptions=Index vector (dialog)  Indices=[1 2]  OutputSizes=1
  Selector1 : Selector  InputPortWidth=3  IndexOptions=Index vector (dialog)  Indices=[1 2]  OutputSizes=1
  Subsystem1 : Subsystem
  Subsystem2 : Subsystem
  Subsystem3 : Subsystem
  Sum : Sum  Inputs=|+-
  Terminator3 : Terminator
  Terminator4 : Terminator
  z_d : Outport
  psi_d : Outport  Port=2
  v : Outport  Port=3
  wires:
  pd(t)'/1 -> Subsystem2/2(pd(t)'), Subsystem1/1(pd(t)'), Selector1/1
  pd(t)/1 -> Derivative/1, Sum/1, Subsystem2/1(pd(t))
  p/1 -> Sum/2, Subsystem2/3(p)
  Subsystem2/1(RTI) -> Matrix Multiply1/1, Display4/1
  2,1/1 -> Mux1/2
  1,1/1 -> Mux1/1
  Subsystem2/3(zd) -> z_d/1
  Gain/1 -> Display/1, psi_d/1
  Subsystem2/2(RWT) -> Matrix Multiply1/2
  Sum/1 -> Display6/1, Scope/1, Selector/1
  Derivative/1 -> Subsystem3/1(In1)
  Subsystem3/1(Out1) -> Scope1/1
  Gain1/1 -> Add1/1
  Add1/1 -> Dot Product1/1
  Mux1/1 -> Dot Product1/2
  Dot Product1/1 -> Display3/1, v/1
  Selector/1 -> Display5/1, Gain1/1
  Selector1/1 -> Add1/2
  Subsystem1/1(Out1) -> Display2/1
  Direction Cosine Matrix to Rotation Angles/1 -> Demux3/1
  Matrix Multiply1/1 -> MATLAB Function/1(u), Display7/1, 2,1/1, 1,1/1
  MATLAB Function/1(y) -> Display1/1, Direction Cosine Matrix to Rotation Angles/1
  Demux3/2 -> Terminator3/1
  Demux3/3 -> Terminator4/1
  Demux3/1 -> Gain/1

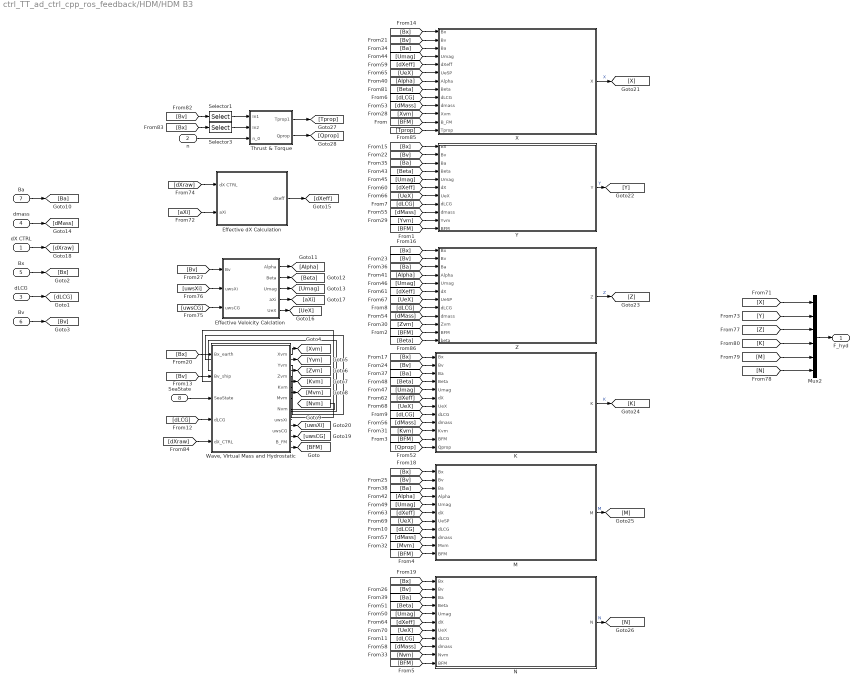
== system ctrl_TT_ad_ctrl_cpp_ros_feedback/HDM/HDM B3 ==
  dX CTRL : Inport
  n : Inport  Port=2
  dLCG : Inport  Port=3
  dmass : Inport  Port=4
  Bx : Inport  Port=5
  Bv : Inport  Port=6
  Ba : Inport  Port=7
  SeaState : Inport  Port=8
  Effective Veloicity Calclation : Subsystem
  Effective dX Calculation : Subsystem
  K : Subsystem
  M : Subsystem
  Mux2 : Mux  Inputs=6
  N : Subsystem
  Selector1 : Selector  InputPortWidth=6  IndexOptions=Index vector (dialog)  Indices=1  OutputSizes=1
  Selector3 : Selector  InputPortWidth=6  IndexOptions=Index vector (dialog)  Indices=3  OutputSizes=1
  Thrust & Torque : Subsystem
  "Wave, Virtual Mass and Hydrostatic" : Subsystem
  X : Subsystem
  Y : Subsystem
  Z : Subsystem
  F_hyd : Outport  VectorParamsAs1DForOutWhenUnconnected=off
  wires:
  Z/1(Z) -> [Z]  "Z"
  [Beta] -> Z/12(beta)
  Thrust & Torque/2(Qprop) -> [Qprop]
  [Tprop] -> X/13(Tprop)
  Thrust & Torque/1(Tprop1) -> [Tprop]
  [Bx] -> Selector3/1
  Selector3/1 -> Thrust & Torque/2(In2)
  Selector1/1 -> Thrust & Torque/1(In1)
  [Bv] -> Selector1/1
  [Qprop] -> K/12(Qprop)
  [N] -> Mux2/6
  [M] -> Mux2/5
  [K] -> Mux2/4
  [Z] -> Mux2/3
  [Y] -> Mux2/2
  [X] -> Mux2/1
  [dXraw] -> "Wave, Virtual Mass and Hydrostatic"/5(dX_CTRL)
  [Beta] -> X/8(Beta)
  N/1(N) -> [N]  "N"
  M/1(M) -> [M]  "M"
  K/1(K) -> [K]  "K"
  Y/1(Y) -> [Y]  "Y"
  X/1(X) -> [X]  "X"
  [uwsXi] -> Effective Veloicity Calclation/2(uwsXi)
  "Wave, Virtual Mass and Hydrostatic"/7(uwsXi) -> [uwsXi]
  [uwsCG] -> Effective Veloicity Calclation/3(uwsCG)
  "Wave, Virtual Mass and Hydrostatic"/8(uwsCG) -> [uwsCG]
  [dXraw] -> Effective dX Calculation/1(dX CTRL)
  dX CTRL/1 -> [dXraw]
  [aXi] -> Effective dX Calculation/2(aXi)
  Effective Veloicity Calclation/4(aXi) -> [aXi]
  [UeX] -> N/7(UeX)
  [UeX] -> M/7(UeSP)
  [UeX] -> K/7(UeX)
  [UeX] -> Z/7(UeSP)
  [UeX] -> Y/7(UeX)
  [UeX] -> X/6(UeSP)
  Effective Veloicity Calclation/5(UeX) -> [UeX]
  [dXeff] -> N/6(dX)
  [dXeff] -> M/6(dX)
  [dXeff] -> K/6(dX)
  [dXeff] -> Z/6(dX)
  [dXeff] -> Y/6(dX)
  [dXeff] -> X/5(dXeff)
  [dMass] -> N/9(dmass)
  [dMass] -> M/9(dmass)
  [dMass] -> K/9(dmass)
  [dMass] -> Y/9(dmass)
  [dMass] -> Z/9(dmass)
  [dMass] -> X/10(dmass)
  dmass/1 -> [dMass]
  [Beta] -> N/4(Beta)
  [Umag] -> N/5(Umag)
  [Umag] -> M/5(Umag)
  [Beta] -> K/4(Beta)
  [Umag] -> K/5(Umag)
  [Umag] -> Z/5(Umag)
  [Umag] -> Y/5(Umag)
  [Umag] -> X/4(Umag)
  Effective Veloicity Calclation/3(Umag) -> [Umag]
  [Beta] -> Y/4(Beta)
  Effective Veloicity Calclation/2(Beta) -> [Beta]
  [Alpha] -> M/4(Alpha)
  [Alpha] -> Z/4(Alpha)
  [Alpha] -> X/7(Alpha)
  Effective Veloicity Calclation/1(Alpha) -> [Alpha]
  [Ba] -> N/3(Ba)
  [Ba] -> M/3(Ba)
  [Ba] -> K/3(Ba)
  [Ba] -> Z/3(Ba)
  [Ba] -> Y/3(Ba)
  [Ba] -> X/3(Ba)
  [Nvm] -> N/10(Nvm)
  [Mvm] -> M/10(Mvm)
  [Kvm] -> K/10(Kvm)
  [Bv] -> Z/2(Bv)
  [Zvm] -> Z/10(Zvm)
  [Yvm] -> Y/10(Yvm)
  [Xvm] -> X/11(Xvm)
  "Wave, Virtual Mass and Hydrostatic"/6(Nvm) -> [Nvm]
  "Wave, Virtual Mass and Hydrostatic"/5(Mvm) -> [Mvm]
  "Wave, Virtual Mass and Hydrostatic"/4(Kvm) -> [Kvm]
  "Wave, Virtual Mass and Hydrostatic"/3(Zvm) -> [Zvm]
  "Wave, Virtual Mass and Hydrostatic"/2(Yvm) -> [Yvm]
  "Wave, Virtual Mass and Hydrostatic"/1(Xvm) -> [Xvm]
  [Bv] -> Effective Veloicity Calclation/1(Bv)
  [Bv] -> N/2(Bv)
  [Bv] -> M/2(Bv)
  [Bv] -> K/2(Bv)
  [Bv] -> Y/2(Bv)
  [Bv] -> X/2(Bv)
  [Bv] -> "Wave, Virtual Mass and Hydrostatic"/2(Bv_ship)
  [Bx] -> "Wave, Virtual Mass and Hydrostatic"/1(Bx_earth)
  [Bx] -> N/1(Bx)
  [Bx] -> M/1(Bx)
  [Bx] -> K/1(Bx)
  [Bx] -> Z/1(Bx)
  [Bx] -> Y/1(Bx)
  [Bx] -> X/1(Bx)
  [dLCG] -> "Wave, Virtual Mass and Hydrostatic"/4(dLCG)
  [dLCG] -> N/8(dLCG)
  [dLCG] -> M/8(dLCG)
  [dLCG] -> K/8(dLCG)
  [dLCG] -> Z/8(dLCG)
  [dLCG] -> Y/8(dLCG)
  [dLCG] -> X/9(dLCG)
  [BFM] -> N/11(BFM)
  [BFM] -> M/11(BFM)
  [BFM] -> K/11(BFM)
  [BFM] -> Z/11(BFM)
  [BFM] -> Y/11(BFM)
  [BFM] -> X/12(B_FM)
  "Wave, Virtual Mass and Hydrostatic"/9(B_FM) -> [BFM]
  n/1 -> Thrust & Torque/3(n_0)
  SeaState/1 -> "Wave, Virtual Mass and Hydrostatic"/3(SeaState)
  Bv/1 -> [Bv]
  dLCG/1 -> [dLCG]
  Bx/1 -> [Bx]
  Ba/1 -> [Ba]
  Effective dX Calculation/1(dXeff) -> [dXeff]
  Mux2/1 -> F_hyd/1

== system ctrl_TT_ad_ctrl_cpp_ros_feedback/HDM/Integration and Coord. Transfrom ==
  Bx : Inport
  F_hyd : Inport  Port=2
  Coordinate Transform : Subsystem
  Rigid Body Motion : Subsystem
  "Bx " : Outport
  Bv : Outport  Port=2
  Ba : Outport  Port=3
  wires:
  Bx/1 -> Rigid Body Motion/2(Bx)
  F_hyd/1 -> Rigid Body Motion/1(F_hyd)
  Rigid Body Motion/2(Ba) -> Ba/1
  Rigid Body Motion/1(Bv) -> Bv/1, Coordinate Transform/1(Bv)
  Coordinate Transform/1(X_earth) -> "Bx "/1

== system ctrl_TT_ad_ctrl_cpp_ros_feedback/HDM/actuator saturation ==
  "dX " : Inport
  "n " : Inport  Port=2
  dLCG : Inport  Port=3
  dmass : Inport  Port=4
  " " : Subsystem
  "   " : Subsystem
  Subsystem1 : Subsystem
  Subsystem2 : Subsystem
  dX : Outport
  n : Outport  Port=2
  dLCG (m) : Outport  Port=3
  dmass (kg) : Outport  Port=4
  wires:
  "n "/1 -> "   "/1("n ")
  Subsystem2/1(dmass (kg)) -> dmass (kg)/1
  "dX "/1 -> " "/1("dX ")
  dmass/1 -> Subsystem2/1(dmass)
  Subsystem1/1(dLCG (m)) -> dLCG (m)/1
  dLCG/1 -> Subsystem1/1(dLCG)
  " "/1(dX) -> dX/1
  "   "/1(n) -> n/1

== system ctrl_TT_ad_ctrl_cpp_ros_feedback/Controller/Subsystem1/Subsystem1 ==
  pd(t)' : Inport
  Add : Sum  Inputs=+++
  Demux : Demux  Outputs=3
  Sqrt : Sqrt
  Square : Math  Operator=square
  Square1 : Math  Operator=square
  Square2 : Math  Operator=square
  Out1 : Outport
  wires:
  Square2/1 -> Add/3
  Demux/3 -> Square2/1
  pd(t)'/1 -> Demux/1
  Demux/1 -> Square/1
  Demux/2 -> Square1/1
  Add/1 -> Sqrt/1
  Square/1 -> Add/1
  Square1/1 -> Add/2
  Sqrt/1 -> Out1/1

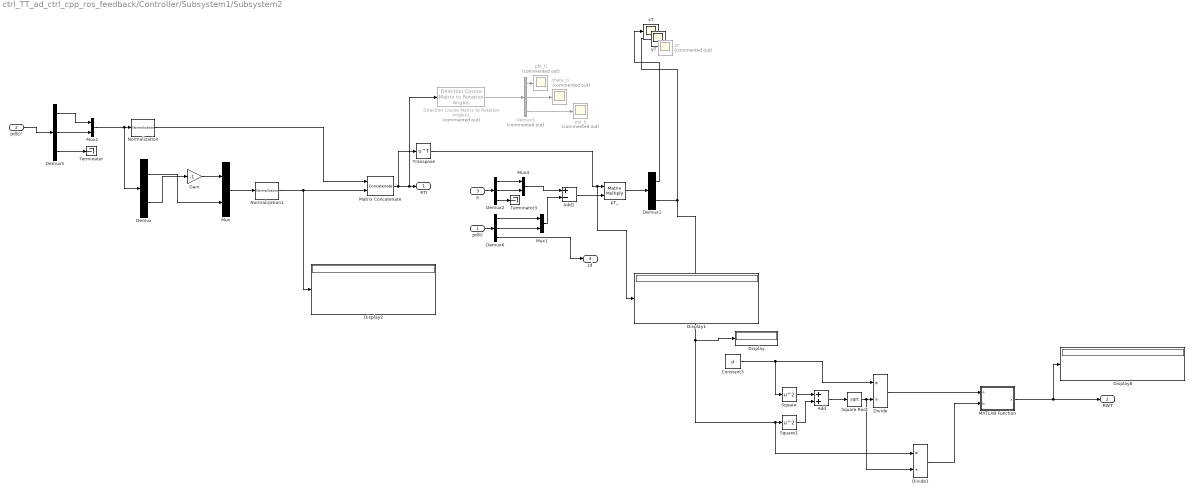
== system ctrl_TT_ad_ctrl_cpp_ros_feedback/Controller/Subsystem1/Subsystem2 ==
  pd(t) : Inport
  pd(t)' : Inport  Port=2
  p : Inport  Port=3
  Add : Sum
  Add1 : Sum  Inputs=+-
  Constant3 : Constant  Value=d
  Demux : Demux  Outputs=2
  Demux1 : Demux  Outputs=2
  Demux2 : Demux  Outputs=3
  Demux3 : Demux  Commented=on  Outputs=3
  Demux5 : Demux  Outputs=3
  Demux6 : Demux  Outputs=3
  Direction Cosine Matrix to Rotation Angles1 : sharedtransform/Direction Cosine Matrix to Rotation Angles  Commented=on  rotationOrder=XYZ  aMode=aMode  action=None  tolerance=eps(2)
  Display{,1..2,8} (4 alike) : Display
  Divide : Product  Inputs=*/
  Divide1 : Product  Inputs=*/
  Gain : Gain  Gain=-1
  MATLAB Function : MATLAB Function  TreatAsAtomicUnit=on
  Matrix Concatenate : Concatenate  Mode=Multidimensional array  ConcatenateDimension=2
  Mux{,1..2,4} (4 alike) : Mux  Inputs=2
  Normalization : dspmathops/Normalization  NormType=2-norm  Bias=1e-10  NormOver=Each column  Dimension=1  roundingMode=Floor  overflowMode=off  accumDataTypeStr=Inherit: Same as product output  accumLastDataTypeStr=Inherit: Same as product output  outputDataTypeStr=Inherit: Same as product output  outputMin=[]  outputMax=[]  outputLastDataTypeStr=Inherit: Same as product output
  Normalization1 : dspmathops/Normalization  NormType=2-norm  Bias=1e-10  NormOver=Each column  Dimension=1  roundingMode=Floor  overflowMode=off  accumDataTypeStr=Inherit: Same as product output  accumLastDataTypeStr=Inherit: Same as product output  outputDataTypeStr=Inherit: Same as product output  outputMin=[]  outputMax=[]  outputLastDataTypeStr=Inherit: Same as product output
  Square : Math  Operator=square
  Square Root : Sqrt
  Square1 : Math  Operator=square
  Terminator : Terminator
  Terminator3 : Terminator
  Transpose : Math  Operator=transpose
  pT_ : Product  Multiplication=Matrix(*)
  phi_ti : Scope  Commented=on
  psi_ti : Scope  Commented=on
  theta_ti : Scope  Commented=on
  xT : Scope
  yT : Scope
  zT : Scope  Commented=on
  RTI : Outport
  RWT : Outport  Port=2
  zd : Outport  Port=3
  wires:
  Gain/1 -> Mux/1
  Demux/2 -> Gain/1
  Demux/1 -> Mux/2
  Mux/1 -> Normalization1/1
  Normalization/1 -> Matrix Concatenate/1
  Normalization1/1 -> Matrix Concatenate/2, Display2/1
  Matrix Concatenate/1 -> Direction Cosine Matrix to Rotation Angles1/1, RTI/1, Transpose/1
  Transpose/1 -> Display1/1, pT_/1
  Add1/1 -> pT_/2
  pT_/1 -> Demux1/1
  Demux1/2 -> yT/1, Display/1, Divide1/1, Square1/1
  Demux1/1 -> xT/1
  Direction Cosine Matrix to Rotation Angles1/1 -> Demux3/1
  Demux3/3 -> psi_ti/1
  Demux3/2 -> theta_ti/1
  Demux3/1 -> phi_ti/1
  Constant3/1 -> Square/1, Divide/1
  Square Root/1 -> Divide1/2, Divide/2
  Add/1 -> Square Root/1
  Square/1 -> Add/1
  Square1/1 -> Add/2
  Divide/1 -> MATLAB Function/1(a)
  Divide1/1 -> MATLAB Function/2(b)
  MATLAB Function/1(y) -> RWT/1, Display8/1
  Demux6/3 -> zd/1
  pd(t)'/1 -> Demux5/1
  Mux2/1 -> Demux/1, Normalization/1
  Demux5/1 -> Mux2/1
  Demux5/2 -> Mux2/2
  Demux5/3 -> Terminator/1
  Demux2/1 -> Mux4/1
  Demux2/3 -> Terminator3/1
  Demux2/2 -> Mux4/2
  Mux4/1 -> Add1/1
  p/1 -> Demux2/1
  Demux6/1 -> Mux1/1
  Demux6/2 -> Mux1/2
  pd(t)/1 -> Demux6/1
  Mux1/1 -> Add1/2

== system ctrl_TT_ad_ctrl_cpp_ros_feedback/Controller/Subsystem1/Subsystem3 ==
  In1 : Inport
  Add : Sum  Inputs=+++
  Demux : Demux  Outputs=3
  Sqrt : Sqrt
  Square : Math  Operator=square
  Square1 : Math  Operator=square
  Square2 : Math  Operator=square
  Out1 : Outport
  wires:
  Sqrt/1 -> Out1/1
  Square1/1 -> Add/2
  Square/1 -> Add/1
  Add/1 -> Sqrt/1
  Demux/2 -> Square1/1
  Demux/1 -> Square/1
  In1/1 -> Demux/1
  Demux/3 -> Square2/1
  Square2/1 -> Add/3

== system ctrl_TT_ad_ctrl_cpp_ros_feedback/HDM/HDM B3/Effective Veloicity Calclation ==
  Bv : Inport
  uwsXi : Inport  Port=2
  uwsCG : Inport  Port=3
  Add{,1..4} (5 alike) : Sum
  Demux : Demux  Outputs=5
  Demux1 : Demux  Outputs=3
  MATLAB Function : MATLAB Function  TreatAsAtomicUnit=on
  MATLAB Function1 : MATLAB Function  TreatAsAtomicUnit=on
  MATLAB Function2 : MATLAB Function  TreatAsAtomicUnit=on
  X_SP1 : Constant  Value=[31.924; 3.861; -3.861;]
  X_SP2 : Constant  Value=[31.924; 3.861; 3.861;]
  X_SP3 : Constant  Value=[31.924; -3.861; 3.861;]
  X_SP4 : Constant  Value=[31.924; -3.861; -3.861;]
  X_XB : Constant  Value=[-10.465; 0; 9.732;]
  n1 : Constant  Value=[0; 1/sqrt(2); -1/sqrt(2);]
  n2 : Constant  Value=[0; 1/sqrt(2); 1/sqrt(2);]
  n3 : Constant  Value=[0; -1/sqrt(2); 1/sqrt(2);]
  n4 : Constant  Value=[0; -1/sqrt(2); -1/sqrt(2);]
  n5 : Constant  Value=[0; 1; 0;]
  nh : Constant  Value=[-1; 0; 0;]
  Alpha : Outport
  Beta : Outport  Port=2
  Umag : Outport  Port=3
  aXi : Outport  Port=4
  UeX : Outport  Port=5
  wires:
  uwsXi/1 -> Demux/1
  MATLAB Function/1(aX) -> aXi/1
  MATLAB Function2/1(alpha) -> Alpha/1
  uwsCG/1 -> Demux1/1
  Demux1/3 -> MATLAB Function2/4(wCG)
  Demux1/2 -> MATLAB Function2/3(vCG)
  Demux1/1 -> MATLAB Function2/2(uCG)
  MATLAB Function/2(UeX) -> UeX/1
  MATLAB Function2/3(Umag) -> Umag/1
  MATLAB Function2/2(beta) -> Beta/1
  MATLAB Function1/2(urX2) -> Add1/1
  MATLAB Function1/3(urX3) -> Add2/1
  MATLAB Function1/4(urX4) -> Add3/1
  MATLAB Function1/5(urXB) -> Add4/1
  Demux/5 -> Add4/2
  Demux/4 -> Add3/2
  Demux/3 -> Add2/2
  Demux/2 -> Add1/2
  Add4/1 -> MATLAB Function/11(urXB)
  Add3/1 -> MATLAB Function/10(urX4)
  Add2/1 -> MATLAB Function/9(urX3)
  Add1/1 -> MATLAB Function/8(urX2)
  Add/1 -> MATLAB Function/7(urX1)
  Demux/1 -> Add/2
  MATLAB Function1/1(urX1) -> Add/1
  n5/1 -> MATLAB Function/6(nB)
  X_SP1/1 -> MATLAB Function1/1(rX1)
  X_SP4/1 -> MATLAB Function1/4(rX4)
  X_SP3/1 -> MATLAB Function1/3(rX3)
  X_SP2/1 -> MATLAB Function1/2(rX2)
  X_XB/1 -> MATLAB Function1/5(rXB)
  n4/1 -> MATLAB Function/5(n4)
  n3/1 -> MATLAB Function/4(n3)
  n2/1 -> MATLAB Function/3(n2)
  n1/1 -> MATLAB Function/2(n1)
  nh/1 -> MATLAB Function/1(nh)
  Bv/1 -> MATLAB Function2/1(Bv), MATLAB Function1/6(U_ship)

== system ctrl_TT_ad_ctrl_cpp_ros_feedback/HDM/HDM B3/Effective dX Calculation ==
  dX CTRL : Inport
  aXi : Inport  Port=2
  Add{,1..4} (5 alike) : Sum
  Demux : Demux  Outputs=5
  Demux1 : Demux  Outputs=5
  Mux6 : Mux  Inputs=5
  dXeff : Outport
  wires:
  Mux6/1 -> dXeff/1
  Demux1/5 -> Add4/2
  Demux1/4 -> Add3/2
  Demux1/3 -> Add2/2
  Demux1/2 -> Add1/2
  Demux1/1 -> Add/2
  Demux/5 -> Add4/1
  Demux/4 -> Add3/1
  Demux/3 -> Add2/1
  Demux/2 -> Add1/1
  Demux/1 -> Add/1
  Add4/1 -> Mux6/5
  Add3/1 -> Mux6/4
  Add2/1 -> Mux6/3
  Add1/1 -> Mux6/2
  Add/1 -> Mux6/1
  aXi/1 -> Demux1/1
  dX CTRL/1 -> Demux/1
